simulink model "WiperSystemControl"  (R2024b)
settings: Solver=FixedStepAuto  StartTime=0.0  StopTime=16  RelTol=1e-3
settings Model: Creator=abhis  LastModifiedBy=abhis
settings DataIOCC: ExternalInput=Sheet1.getElement('WiprMod'),Sheet1.getElement('WiprSpdReq'),Sheet1.getElement('RainSnsrErr')  LoadExternalInput=on

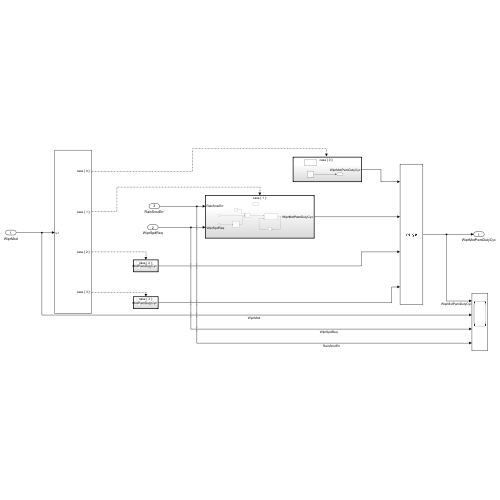
[thumbnail: Simulink's stored preview of the top-level diagram]
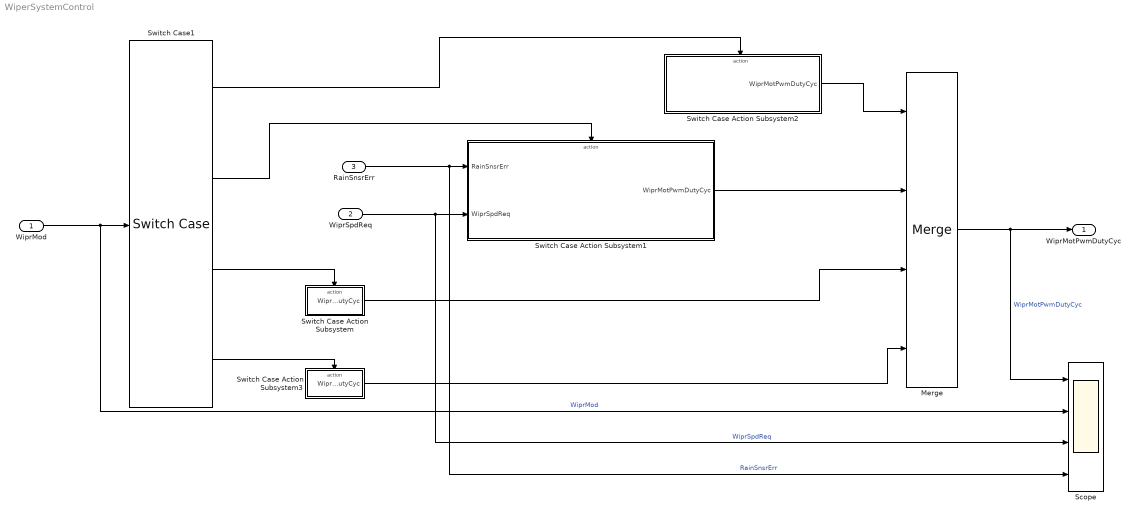
== system WiperSystemControl ==
  WiprMod : Inport  OutDataTypeStr=uint8
  WiprSpdReq : Inport  Port=2  OutDataTypeStr=single
  RainSnsrErr : Inport  Port=3  OutDataTypeStr=boolean
  Merge : Merge  Inputs=4  InitialOutput=0
  Scope : Scope  NumInputPorts=4
  Switch Case Action Subsystem : Subsystem  TreatAsAtomicUnit=on
  Switch Case Action Subsystem1 : Subsystem  TreatAsAtomicUnit=on
  Switch Case Action Subsystem2 : Subsystem  TreatAsAtomicUnit=on
  Switch Case Action Subsystem3 : Subsystem  TreatAsAtomicUnit=on
  Switch Case1 : SwitchCase  CaseConditions={0,1,2,3}  ShowDefaultCase=off
  WiprMotPwmDutyCyc : Outport
  wires:
  Switch Case Action Subsystem2/1(WiprMotPwmDutyCyc) -> Merge/1
  Switch Case Action Subsystem3/1(WiprMotPwmDutyCyc) -> Merge/4
  Switch Case Action Subsystem/1(WiprMotPwmDutyCyc) -> Merge/3
  Merge/1 -> Scope/1, WiprMotPwmDutyCyc/1  "WiprMotPwmDutyCyc"
  RainSnsrErr/1 -> Scope/4, Switch Case Action Subsystem1/1(RainSnsrErr)  "RainSnsrErr"
  WiprSpdReq/1 -> Scope/3, Switch Case Action Subsystem1/2(WiprSpdReq)  "WiprSpdReq"
  Switch Case Action Subsystem1/1(WiprMotPwmDutyCyc) -> Merge/2
  Switch Case1/4 -> Switch Case Action Subsystem3/Action
  Switch Case1/3 -> Switch Case Action Subsystem/Action
  Switch Case1/2 -> Switch Case Action Subsystem1/Action
  Switch Case1/1 -> Switch Case Action Subsystem2/Action
  WiprMod/1 -> Scope/2, Switch Case1/1  "WiprMod"

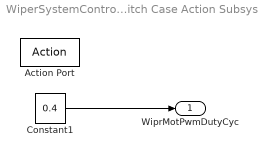
== system WiperSystemControl/Switch Case Action Subsystem ==
  Action Port : ActionPort  ActionPortLabel=case [ 2 ]:
  Constant1 : Constant  Value=0.4  OutDataTypeStr=Inherit: Inherit via back propagation
  WiprMotPwmDutyCyc : Outport
  wires:
  Constant1/1 -> WiprMotPwmDutyCyc/1

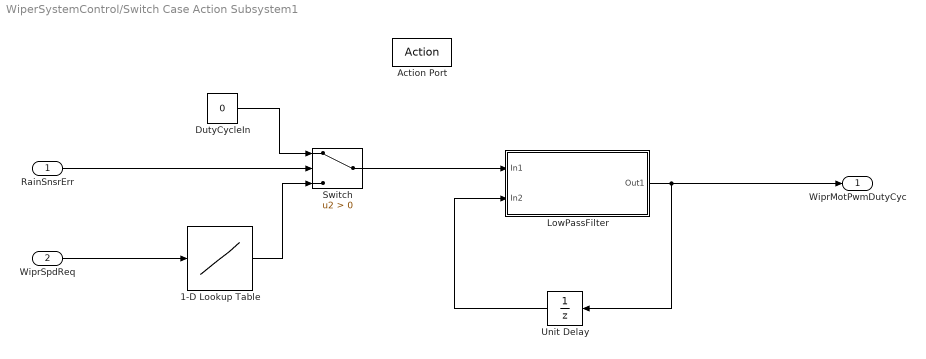
== system WiperSystemControl/Switch Case Action Subsystem1 ==
  RainSnsrErr : Inport  OutDataTypeStr=boolean
  WiprSpdReq : Inport  Port=2  OutDataTypeStr=single
  Action Port : ActionPort  ActionPortLabel=case [ 1 ]:
  1-D Lookup Table : Lookup_n-D  NumberOfTableDimensions=1  BreakpointsForDimension1=[0;1;2;3;4;5;6;7]  Table=[0;0.40;0.45;0.50;0.55;0.60;0.65;0.70]  TableDataTypeStr=single  InternalRulePriority=Speed  OutDataTypeStr=single  RndMeth=Simplest
  DutyCycleIn : Constant  Value=0  OutDataTypeStr=single
  LowPassFilter : Subsystem
  Switch : Switch  Criteria=u2 > Threshold  OutDataTypeStr=single  SaturateOnIntegerOverflow=off  InputSameDT=off
  Unit Delay : UnitDelay  SampleTime=-1  HasFrameUpgradeWarning=on
  WiprMotPwmDutyCyc : Outport  OutDataTypeStr=single
  wires:
  WiprSpdReq/1 -> 1-D Lookup Table/1
  Switch/1 -> LowPassFilter/1(In1)
  Unit Delay/1 -> LowPassFilter/2(In2)
  1-D Lookup Table/1 -> Switch/3
  DutyCycleIn/1 -> Switch/1
  LowPassFilter/1(Out1) -> WiprMotPwmDutyCyc/1, Unit Delay/1
  RainSnsrErr/1 -> Switch/2

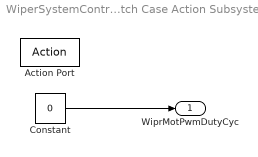
== system WiperSystemControl/Switch Case Action Subsystem2 ==
  Action Port : ActionPort  ActionPortLabel=case [ 0 ]:
  Constant : Constant  Value=0  OutDataTypeStr=Inherit: Inherit via back propagation
  WiprMotPwmDutyCyc : Outport
  wires:
  Constant/1 -> WiprMotPwmDutyCyc/1

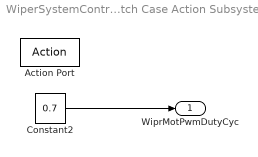
== system WiperSystemControl/Switch Case Action Subsystem3 ==
  Action Port : ActionPort  ActionPortLabel=case [ 3 ]:
  Constant2 : Constant  Value=0.7  OutDataTypeStr=Inherit: Inherit via back propagation
  WiprMotPwmDutyCyc : Outport
  wires:
  Constant2/1 -> WiprMotPwmDutyCyc/1

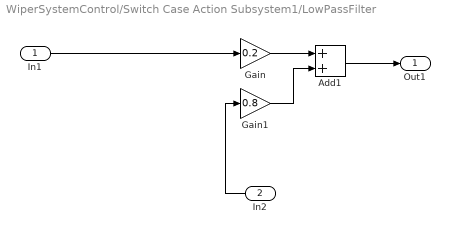
== system WiperSystemControl/Switch Case Action Subsystem1/LowPassFilter ==
  In1 : Inport
  In2 : Inport  Port=2
  Add1 : Sum
  Gain : Gain  Gain=0.2
  Gain1 : Gain  Gain=0.8
  Out1 : Outport
  wires:
  In1/1 -> Gain/1
  Gain/1 -> Add1/1
  Gain1/1 -> Add1/2
  In2/1 -> Gain1/1
  Add1/1 -> Out1/1
